simulink model "Muscles_6DOFMuscle"  (R2021b)
settings: Solver=VariableStepAuto  StartTime=0.0  StopTime=10.0  RelTol=1e-3
values from neighbouring files (symbols this model uses):
  N = length(dataset.(fldnames{1}))    [create_timeseries.m]    (also in input_data.m = length(t); test_input_data.m = length(t))
  Param_Mus_MEE = Library_mtu_simulink_mtu_standard_parameters(Param_Mus_MEE)    [init_muscle_MEE.m]
  Param_Mus_MEF = Library_mtu_simulink_mtu_standard_parameters(Param_Mus_MEF)    [init_muscle_MEF.m]
undefined symbols (not defined in the file or in its folder): gen_param
libraries: Library_mtu_simulink x12, nesl_utility x9, sm_lib x1
settings Model: Creator=Strel  LastModifiedBy=Strel

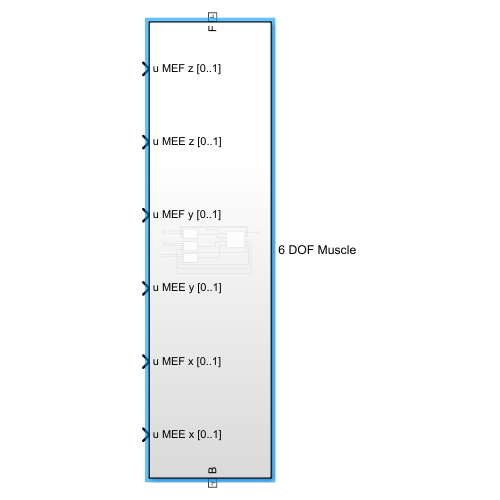
[thumbnail: Simulink's stored preview of the top-level diagram]
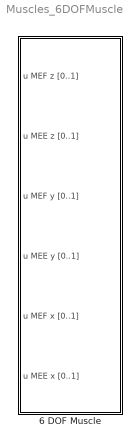
== system Muscles_6DOFMuscle ==
  6 DOF Muscle : Subsystem
      settings: PortSchema="{\"entries\":[{\"content\":{\"sides\":[{\"content\":{\"connectorIds\":[\"LConn1\"]},\"type\":\"ConnectorPlacement.EquallySpacedRectSide\",\"uuid\":\"c57921d5-7669-4cd5-a2e2-a585923a98fb\"},{\"content\":{\"connectorIds\":[\"RConn1\"],\"side\":\"RIGHT\"},\"type\":\"ConnectorPlacement.EquallySpacedRectSide\",\"uuid\":\"a6a62461-cd3b-465b-b4ac-8ccaada5b936\"},{\"content\":{\"connectorIds\":[\"In1\",\"In2\",\"In3\",\"In4\",\"In5\",\"In6\"],\"side\":\"TOP\"},\"type\":\"ConnectorPlacement.EquallySpacedRectSide\",\"uuid\":\"09a39f01-a3c0-4da8-ba68-41ece68877e3\"}]},\"type\":\"ConnectorPlacement.EquallySpacedConnector\",\"uuid\":\"fc42cfe5-3873-4c4a-917f-8e9d216a7f60\"}],\"packageUris\":[\"http://schema.mathworks.com/mf0/Connector/R2020b\"],\"version\":\"1.0\"}"

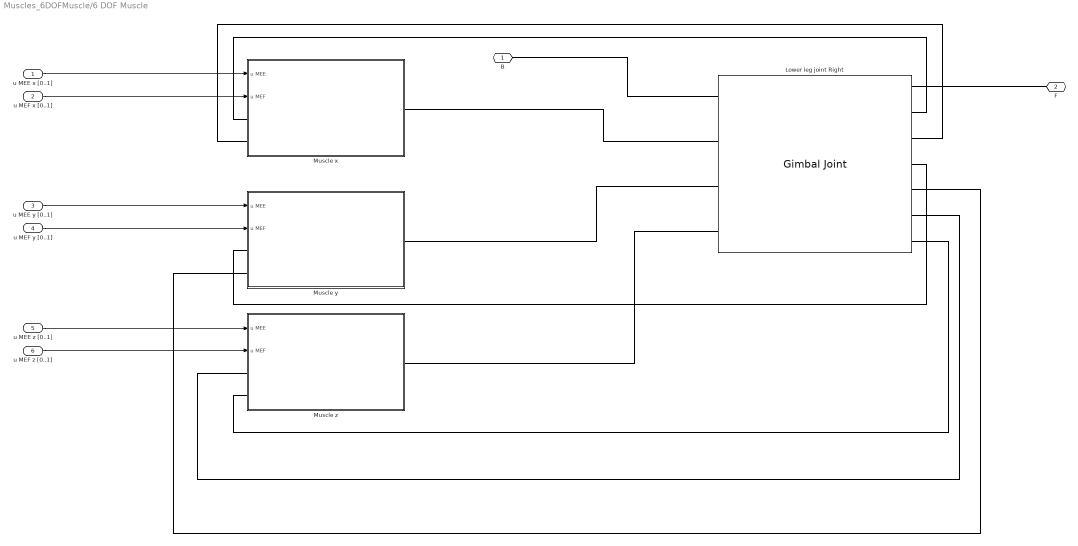
== system Muscles_6DOFMuscle/6 DOF Muscle ==
  u MEE x [0..1] : Inport
  u MEF x [0..1] : Inport  Port=2
  u MEE y [0..1] : Inport  Port=3
  u MEF y [0..1] : Inport  Port=4
  u MEE z [0..1] : Inport  Port=5
  u MEF z [0..1] : Inport  Port=6
  Lower leg joint Right : sm_lib/Joints/Gimbal Joint  JointMode=Normal  SenseConstraintForce=off  SenseConstraintForceX=off  SenseConstraintForceY=off  SenseConstraintForceZ=off  SenseConstraintTorque=off  SenseConstraintTorqueX=off  SenseConstraintTorqueY=off  SenseConstraintTorqueZ=off  SenseTotalForce=off  SenseTotalForceX=off  SenseTotalForceY=off  SenseTotalForceZ=off  SenseTotalTorque=off  SenseTotalTorqueX=off  SenseTotalTorqueY=off  SenseTotalTorqueZ=off  CompositeWrenchDir=FollowerOnBase  CompositeWrenchFrame=BaseFrame  RxEquilibriumPosition=0  RxEquilibriumPositionUnits=deg  RxSpringStiffness=0  RxSpringStiffnessUnits=N*m/deg  RxDampingCoefficient=0  RxDampingCoefficientUnits=N*m/(deg/s)  RxTorqueActuationMode=InputTorque  RxMotionActuationMode=ComputedMotion  RxSensePosition=on  RxSenseVelocity=on  RxSenseAcceleration=off  RxSenseTorqueForce=off  RxSenseLowerLimitTorqueForce=off  RxSenseUpperLimitTorqueForce=off  RxLowerLimitSpecify=on  RxLowerLimitBound=-90  RxLowerLimitBoundUnits=deg  RxLowerLimitStiffness=bodyparam.stiffness.femur  RxLowerLimitStiffnessUnits=N*m/deg  RxLowerLimitDamping=bodyparam.damping.femur  RxLowerLimitDampingUnits=N*m/(deg/s)  RxLowerLimitTransitionRegionWidth=0.1  RxLowerLimitTransitionRegionWidthUnits=deg  RxUpperLimitSpecify=on  RxUpperLimitBound=90  RxUpperLimitBoundUnits=deg  RxUpperLimitStiffness=bodyparam.stiffness.femur  RxUpperLimitStiffnessUnits=N*m/rad  RxUpperLimitDamping=bodyparam.damping.femur  RxUpperLimitDampingUnits=N*m/(rad/s)  RxUpperLimitTransitionRegionWidth=0.1  RxUpperLimitTransitionRegionWidthUnits=deg  RxPositionTargetSpecify=off  RxPositionTargetPriority=High  RxPositionTargetValue=0  RxPositionTargetValueUnits=deg  RxVelocityTargetSpecify=off  RxVelocityTargetPriority=High  RxVelocityTargetValue=0  RxVelocityTargetValueUnits=deg/s  RyEquilibriumPosition=0  RyEquilibriumPositionUnits=deg  RySpringStiffness=0  RySpringStiffnessUnits=N*m/deg  RyDampingCoefficient=0  RyDampingCoefficientUnits=N*m/(deg/s)  RyTorqueActuationMode=InputTorque  RyMotionActuationMode=ComputedMotion  RySensePosition=on  RySenseVelocity=on  RySenseAcceleration=off  RySenseTorqueForce=off  RySenseLowerLimitTorqueForce=off  RySenseUpperLimitTorqueForce=off  RyLowerLimitSpecify=on  RyLowerLimitBound=0  RyLowerLimitBoundUnits=deg  RyLowerLimitStiffness=bodyparam.stiffness.femur  RyLowerLimitStiffnessUnits=N*m/rad  RyLowerLimitDamping=bodyparam.damping.femur  RyLowerLimitDampingUnits=N*m/(rad/s)  RyLowerLimitTransitionRegionWidth=0.1  RyLowerLimitTransitionRegionWidthUnits=deg  RyUpperLimitSpecify=on  RyUpperLimitBound=90  RyUpperLimitBoundUnits=deg  RyUpperLimitStiffness=bodyparam.stiffness.femur  RyUpperLimitStiffnessUnits=N*m/rad  RyUpperLimitDamping=bodyparam.damping.femur  RyUpperLimitDampingUnits=N*m/(rad/s)  RyUpperLimitTransitionRegionWidth=0.1  RyUpperLimitTransitionRegionWidthUnits=deg  RyPositionTargetSpecify=off  RyPositionTargetPriority=High  RyPositionTargetValue=0  RyPositionTargetValueUnits=deg  RyVelocityTargetSpecify=off  RyVelocityTargetPriority=High  RyVelocityTargetValue=0  RyVelocityTargetValueUnits=deg/s  RzEquilibriumPosition=0  RzEquilibriumPositionUnits=deg  RzSpringStiffness=0  RzSpringStiffnessUnits=N*m/deg  RzDampingCoefficient=0  RzDampingCoefficientUnits=N*m/(deg/s)  RzTorqueActuationMode=InputTorque  RzMotionActuationMode=ComputedMotion  RzSensePosition=on  RzSenseVelocity=on  RzSenseAcceleration=off  RzSenseTorqueForce=off  RzSenseLowerLimitTorqueForce=off  RzSenseUpperLimitTorqueForce=off  RzLowerLimitSpecify=on  RzLowerLimitBound=-90  RzLowerLimitBoundUnits=deg  RzLowerLimitStiffness=bodyparam.stiffness.femur  RzLowerLimitStiffnessUnits=N*m/rad  RzLowerLimitDamping=bodyparam.damping.femur  RzLowerLimitDampingUnits=N*m/(rad/s)  RzLowerLimitTransitionRegionWidth=0.1  RzLowerLimitTransitionRegionWidthUnits=deg  RzUpperLimitSpecify=on  RzUpperLimitBound=90  RzUpperLimitBoundUnits=deg  RzUpperLimitStiffness=bodyparam.stiffness.femur  RzUpperLimitStiffnessUnits=N*m/rad  RzUpperLimitDamping=bodyparam.damping.femur  RzUpperLimitDampingUnits=N*m/(rad/s)  RzUpperLimitTransitionRegionWidth=0.1  RzUpperLimitTransitionRegionWidthUnits=deg  RzPositionTargetSpecify=off  RzPositionTargetPriority=High  RzPositionTargetValue=0  RzPositionTargetValueUnits=deg  RzVelocityTargetSpecify=off  RzVelocityTargetPriority=High  RzVelocityTargetValue=0  RzVelocityTargetValueUnits=deg/s
  Muscle x : Subsystem
  Muscle y : Subsystem
  Muscle z : Subsystem
  B : PMIOPort  Side=Left
  F : PMIOPort  Port=2  Side=Right
  wires:
  u MEE x [0..1]/1 -> Muscle x/1(u MEE)
  u MEF x [0..1]/1 -> Muscle x/2(u MEF)
  u MEF y [0..1]/1 -> Muscle y/2(u MEF)
  u MEE y [0..1]/1 -> Muscle y/1(u MEE)
  u MEF z [0..1]/1 -> Muscle z/2(u MEF)
  u MEE z [0..1]/1 -> Muscle z/1(u MEE)
  connections:
  B/RConn1 -- Lower leg joint Right/LConn1
  F/RConn1 -- Lower leg joint Right/RConn1
  Muscle x/RConn1 -- Lower leg joint Right/LConn2
  Muscle y/RConn1 -- Lower leg joint Right/LConn3
  Muscle z/RConn1 -- Lower leg joint Right/LConn4
  Lower leg joint Right/RConn2 -- Muscle x/LConn1
  Muscle x/LConn2 -- Lower leg joint Right/RConn3
  Lower leg joint Right/RConn4 -- Muscle y/LConn1
  Lower leg joint Right/RConn5 -- Muscle y/LConn2
  Lower leg joint Right/RConn6 -- Muscle z/LConn1
  Lower leg joint Right/RConn7 -- Muscle z/LConn2

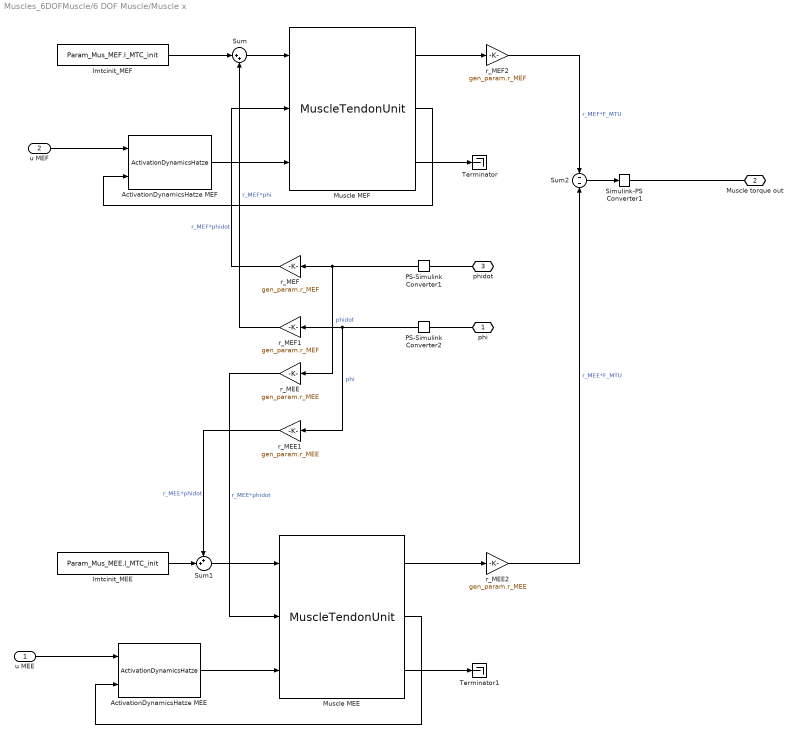
== system Muscles_6DOFMuscle/6 DOF Muscle/Muscle x ==
  u MEE : Inport
  u MEF : Inport  Port=2
  ActivationDynamicsHatze MEE : Library_mtu_simulink/ActivationDynamicsHatze  Act_Param=Param_Mus_MEE.ActDyn  Mus_Param=Param_Mus_MEE
  ActivationDynamicsHatze MEF : Library_mtu_simulink/ActivationDynamicsHatze  Act_Param=Param_Mus_MEF.ActDyn  Mus_Param=Param_Mus_MEF
  Imtcinit_MEE : Constant  Value=Param_Mus_MEE.l_MTC_init
  Imtcinit_MEF : Constant  Value=Param_Mus_MEF.l_MTC_init
  Muscle MEE : Library_mtu_simulink/MuscleTendonUnit  Mus_Param=Param_Mus_MEE
  Muscle MEF : Library_mtu_simulink/MuscleTendonUnit  Mus_Param=Param_Mus_MEF
  PS-Simulink Converter1 : nesl_utility/PS-Simulink Converter  PhysicalDomain=network_engine_domain  SubClassName=ps_output  LeftPortType=input  RightPortType=output  PseudoPeriodic=off  Frequencies=[]  Unit=inherit  AffineConversion=off
      settings: SourceProductBaseCode=PW,SS
  PS-Simulink Converter2 : nesl_utility/PS-Simulink Converter  PhysicalDomain=network_engine_domain  SubClassName=ps_output  LeftPortType=input  RightPortType=output  PseudoPeriodic=off  Frequencies=[]  Unit=inherit  AffineConversion=off
      settings: SourceProductBaseCode=PW,SS
  Simulink-PS Converter1 : nesl_utility/Simulink-PS Converter  PhysicalDomain=network_engine_domain  SubClassName=ps_input  LeftPortType=input  RightPortType=output  PseudoPeriodic=off  Frequencies=[]  NoiseDistribution=none  NoiseParameters=[]  Unit=1  AffineConversion=off  FilteringAndDerivatives=provide  SimscapeFilterOrder=1  InputFilterTimeConstant=0.001  UdotUserProvided=0
      settings: SourceProductBaseCode=PW,SS
  Sum : Sum  Inputs=|++
  Sum1 : Sum  Inputs=++|
  Sum2 : Sum  Inputs=--
  Terminator : Terminator
  Terminator1 : Terminator
  r_MEE : Gain  Gain=gen_param.r_MEE
  r_MEE1 : Gain  Gain=gen_param.r_MEE
  r_MEE2 : Gain  Gain=gen_param.r_MEE
  r_MEF : Gain  Gain=gen_param.r_MEF
  r_MEF1 : Gain  Gain=gen_param.r_MEF
  r_MEF2 : Gain  Gain=gen_param.r_MEF
  phi : PMIOPort  Side=Left
  Muscle torque out : PMIOPort  Port=2  Side=Right
  phidot : PMIOPort  Port=3  Side=Left
  wires:
  r_MEF1/1 -> Sum/2  "r_MEF*phi"
  u MEE/1 -> ActivationDynamicsHatze MEE/1
  r_MEE1/1 -> Sum1/1  "r_MEE*phidot"
  Sum1/1 -> Muscle MEE/1
  u MEF/1 -> ActivationDynamicsHatze MEF/1
  Muscle MEF/2 -> ActivationDynamicsHatze MEF/2
  Muscle MEF/1 -> r_MEF2/1
  Muscle MEE/2 -> ActivationDynamicsHatze MEE/2
  ActivationDynamicsHatze MEF/1 -> Muscle MEF/3
  PS-Simulink Converter1/1 -> r_MEE/1, r_MEF/1  "phidot"
  Sum/1 -> Muscle MEF/1
  Muscle MEE/1 -> r_MEE2/1
  ActivationDynamicsHatze MEE/1 -> Muscle MEE/3
  Imtcinit_MEF/1 -> Sum/1
  r_MEF/1 -> Muscle MEF/2  "r_MEF*phidot"
  PS-Simulink Converter2/1 -> r_MEE1/1, r_MEF1/1  "phi"
  Sum2/1 -> Simulink-PS Converter1/1
  Muscle MEF/3 -> Terminator/1
  Muscle MEE/3 -> Terminator1/1
  Imtcinit_MEE/1 -> Sum1/2
  r_MEE/1 -> Muscle MEE/2  "r_MEE*phidot"
  r_MEE2/1 -> Sum2/2  "r_MEE*F_MTU"
  r_MEF2/1 -> Sum2/1  "r_MEF*F_MTU"
  connections:
  PS-Simulink Converter2/LConn1 -- phi/RConn1
  PS-Simulink Converter1/LConn1 -- phidot/RConn1
  Simulink-PS Converter1/RConn1 -- Muscle torque out/RConn1

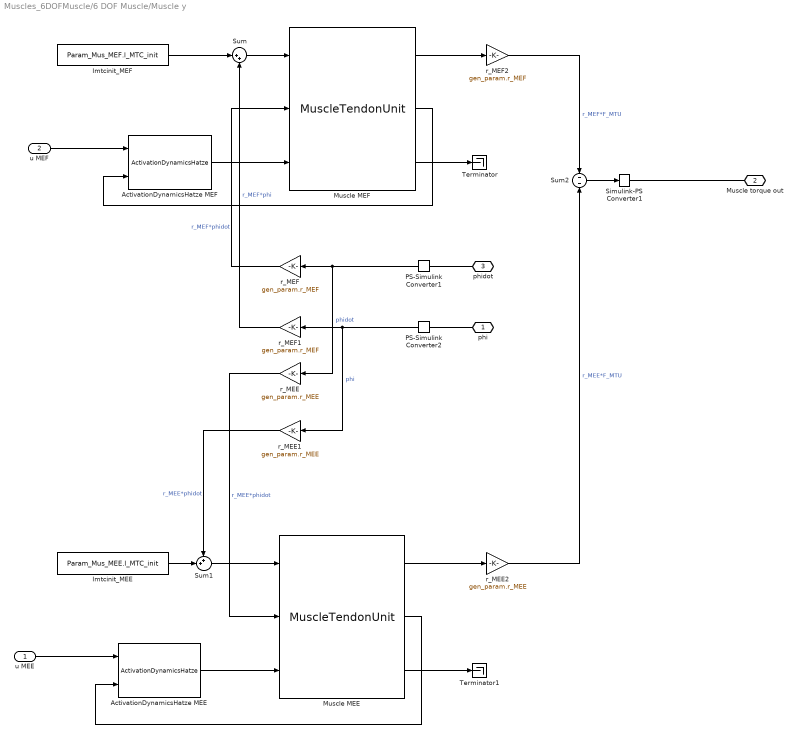
== system Muscles_6DOFMuscle/6 DOF Muscle/Muscle y ==
  u MEE : Inport
  u MEF : Inport  Port=2
  ActivationDynamicsHatze MEE : Library_mtu_simulink/ActivationDynamicsHatze  Act_Param=Param_Mus_MEE.ActDyn  Mus_Param=Param_Mus_MEE
  ActivationDynamicsHatze MEF : Library_mtu_simulink/ActivationDynamicsHatze  Act_Param=Param_Mus_MEF.ActDyn  Mus_Param=Param_Mus_MEF
  Imtcinit_MEE : Constant  Value=Param_Mus_MEE.l_MTC_init
  Imtcinit_MEF : Constant  Value=Param_Mus_MEF.l_MTC_init
  Muscle MEE : Library_mtu_simulink/MuscleTendonUnit  Mus_Param=Param_Mus_MEE
  Muscle MEF : Library_mtu_simulink/MuscleTendonUnit  Mus_Param=Param_Mus_MEF
  PS-Simulink Converter1 : nesl_utility/PS-Simulink Converter  PhysicalDomain=network_engine_domain  SubClassName=ps_output  LeftPortType=input  RightPortType=output  PseudoPeriodic=off  Frequencies=[]  Unit=inherit  AffineConversion=off
      settings: SourceProductBaseCode=PW,SS
  PS-Simulink Converter2 : nesl_utility/PS-Simulink Converter  PhysicalDomain=network_engine_domain  SubClassName=ps_output  LeftPortType=input  RightPortType=output  PseudoPeriodic=off  Frequencies=[]  Unit=inherit  AffineConversion=off
      settings: SourceProductBaseCode=PW,SS
  Simulink-PS Converter1 : nesl_utility/Simulink-PS Converter  PhysicalDomain=network_engine_domain  SubClassName=ps_input  LeftPortType=input  RightPortType=output  PseudoPeriodic=off  Frequencies=[]  NoiseDistribution=none  NoiseParameters=[]  Unit=1  AffineConversion=off  FilteringAndDerivatives=provide  SimscapeFilterOrder=1  InputFilterTimeConstant=0.001  UdotUserProvided=0
      settings: SourceProductBaseCode=PW,SS
  Sum : Sum  Inputs=|++
  Sum1 : Sum  Inputs=++|
  Sum2 : Sum  Inputs=--
  Terminator : Terminator
  Terminator1 : Terminator
  r_MEE : Gain  Gain=gen_param.r_MEE
  r_MEE1 : Gain  Gain=gen_param.r_MEE
  r_MEE2 : Gain  Gain=gen_param.r_MEE
  r_MEF : Gain  Gain=gen_param.r_MEF
  r_MEF1 : Gain  Gain=gen_param.r_MEF
  r_MEF2 : Gain  Gain=gen_param.r_MEF
  phi : PMIOPort  Side=Left
  Muscle torque out : PMIOPort  Port=2  Side=Right
  phidot : PMIOPort  Port=3  Side=Left
  wires:
  r_MEF1/1 -> Sum/2  "r_MEF*phi"
  u MEE/1 -> ActivationDynamicsHatze MEE/1
  r_MEE1/1 -> Sum1/1  "r_MEE*phidot"
  Sum1/1 -> Muscle MEE/1
  u MEF/1 -> ActivationDynamicsHatze MEF/1
  Muscle MEF/2 -> ActivationDynamicsHatze MEF/2
  Muscle MEF/1 -> r_MEF2/1
  Muscle MEE/2 -> ActivationDynamicsHatze MEE/2
  ActivationDynamicsHatze MEF/1 -> Muscle MEF/3
  PS-Simulink Converter1/1 -> r_MEE/1, r_MEF/1  "phidot"
  Sum/1 -> Muscle MEF/1
  Muscle MEE/1 -> r_MEE2/1
  ActivationDynamicsHatze MEE/1 -> Muscle MEE/3
  Imtcinit_MEF/1 -> Sum/1
  r_MEF/1 -> Muscle MEF/2  "r_MEF*phidot"
  PS-Simulink Converter2/1 -> r_MEE1/1, r_MEF1/1  "phi"
  Sum2/1 -> Simulink-PS Converter1/1
  Muscle MEF/3 -> Terminator/1
  Muscle MEE/3 -> Terminator1/1
  Imtcinit_MEE/1 -> Sum1/2
  r_MEE/1 -> Muscle MEE/2  "r_MEE*phidot"
  r_MEE2/1 -> Sum2/2  "r_MEE*F_MTU"
  r_MEF2/1 -> Sum2/1  "r_MEF*F_MTU"
  connections:
  PS-Simulink Converter2/LConn1 -- phi/RConn1
  PS-Simulink Converter1/LConn1 -- phidot/RConn1
  Simulink-PS Converter1/RConn1 -- Muscle torque out/RConn1

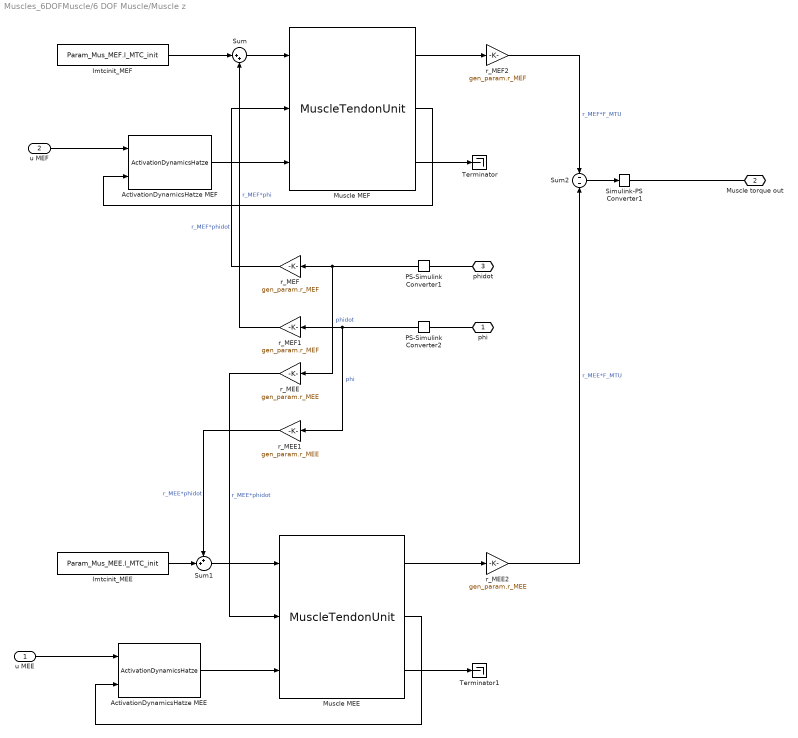
== system Muscles_6DOFMuscle/6 DOF Muscle/Muscle z ==
  u MEE : Inport
  u MEF : Inport  Port=2
  ActivationDynamicsHatze MEE : Library_mtu_simulink/ActivationDynamicsHatze  Act_Param=Param_Mus_MEE.ActDyn  Mus_Param=Param_Mus_MEE
  ActivationDynamicsHatze MEF : Library_mtu_simulink/ActivationDynamicsHatze  Act_Param=Param_Mus_MEF.ActDyn  Mus_Param=Param_Mus_MEF
  Imtcinit_MEE : Constant  Value=Param_Mus_MEE.l_MTC_init
  Imtcinit_MEF : Constant  Value=Param_Mus_MEF.l_MTC_init
  Muscle MEE : Library_mtu_simulink/MuscleTendonUnit  Mus_Param=Param_Mus_MEE
  Muscle MEF : Library_mtu_simulink/MuscleTendonUnit  Mus_Param=Param_Mus_MEF
  PS-Simulink Converter1 : nesl_utility/PS-Simulink Converter  PhysicalDomain=network_engine_domain  SubClassName=ps_output  LeftPortType=input  RightPortType=output  PseudoPeriodic=off  Frequencies=[]  Unit=inherit  AffineConversion=off
      settings: SourceProductBaseCode=PW,SS
  PS-Simulink Converter2 : nesl_utility/PS-Simulink Converter  PhysicalDomain=network_engine_domain  SubClassName=ps_output  LeftPortType=input  RightPortType=output  PseudoPeriodic=off  Frequencies=[]  Unit=inherit  AffineConversion=off
      settings: SourceProductBaseCode=PW,SS
  Simulink-PS Converter1 : nesl_utility/Simulink-PS Converter  PhysicalDomain=network_engine_domain  SubClassName=ps_input  LeftPortType=input  RightPortType=output  PseudoPeriodic=off  Frequencies=[]  NoiseDistribution=none  NoiseParameters=[]  Unit=1  AffineConversion=off  FilteringAndDerivatives=provide  SimscapeFilterOrder=1  InputFilterTimeConstant=0.001  UdotUserProvided=0
      settings: SourceProductBaseCode=PW,SS
  Sum : Sum  Inputs=|++
  Sum1 : Sum  Inputs=++|
  Sum2 : Sum  Inputs=--
  Terminator : Terminator
  Terminator1 : Terminator
  r_MEE : Gain  Gain=gen_param.r_MEE
  r_MEE1 : Gain  Gain=gen_param.r_MEE
  r_MEE2 : Gain  Gain=gen_param.r_MEE
  r_MEF : Gain  Gain=gen_param.r_MEF
  r_MEF1 : Gain  Gain=gen_param.r_MEF
  r_MEF2 : Gain  Gain=gen_param.r_MEF
  phi : PMIOPort  Side=Left
  Muscle torque out : PMIOPort  Port=2  Side=Right
  phidot : PMIOPort  Port=3  Side=Left
  wires:
  r_MEF1/1 -> Sum/2  "r_MEF*phi"
  u MEE/1 -> ActivationDynamicsHatze MEE/1
  r_MEE1/1 -> Sum1/1  "r_MEE*phidot"
  Sum1/1 -> Muscle MEE/1
  u MEF/1 -> ActivationDynamicsHatze MEF/1
  Muscle MEF/2 -> ActivationDynamicsHatze MEF/2
  Muscle MEF/1 -> r_MEF2/1
  Muscle MEE/2 -> ActivationDynamicsHatze MEE/2
  ActivationDynamicsHatze MEF/1 -> Muscle MEF/3
  PS-Simulink Converter1/1 -> r_MEE/1, r_MEF/1  "phidot"
  Sum/1 -> Muscle MEF/1
  Muscle MEE/1 -> r_MEE2/1
  ActivationDynamicsHatze MEE/1 -> Muscle MEE/3
  Imtcinit_MEF/1 -> Sum/1
  r_MEF/1 -> Muscle MEF/2  "r_MEF*phidot"
  PS-Simulink Converter2/1 -> r_MEE1/1, r_MEF1/1  "phi"
  Sum2/1 -> Simulink-PS Converter1/1
  Muscle MEF/3 -> Terminator/1
  Muscle MEE/3 -> Terminator1/1
  Imtcinit_MEE/1 -> Sum1/2
  r_MEE/1 -> Muscle MEE/2  "r_MEE*phidot"
  r_MEE2/1 -> Sum2/2  "r_MEE*F_MTU"
  r_MEF2/1 -> Sum2/1  "r_MEF*F_MTU"
  connections:
  PS-Simulink Converter2/LConn1 -- phi/RConn1
  PS-Simulink Converter1/LConn1 -- phidot/RConn1
  Simulink-PS Converter1/RConn1 -- Muscle torque out/RConn1
